simulink model "net"  (R2018a)
settings: Solver=VariableStepAuto  StartTime=0.0  StopTime=10.0  RelTol=1e-3
libraries: neural x115
(part 6 of 6)

== system net/Function Fitting Neural Network/Layer 5/Delays 1 ==
  "p{5}" : Inport  PortDimensions=30
      mask Display: e = 0.06;c1 = [120 230 180]/255;c2 = ([120 230 180]+0)/(256+128);c3 = ([120 230 180]+128)/(256+128);patch([0 1 1 0],[0 0 1 1],c1);patch([0 1 1 1-e 1-e 0+e],[0 0 1 1-e 0+e 0+e],c2);patch([0 0 1 1-e 0+e 0+e],[0 1 1 1-e 1-e 0+e],c3);plot([0 1 1 0 0],[0 0 1 1 0]);
  mux : Mux  Inputs=1
      mask Display: e = 0.06;c1 = [120 150 230]/255;c2 = ([120 150 230]+0)/383;c3 = ([120 150 230]+128)/383;patch([0 1 1 0],[0 0 1 1],c1);patch([0 1 1 1-e 1-e 0+e],[0 0 1 1-e 0+e 0+e],c2);patch([0 0 1 1-e 0+e 0+e],[0 1 1 1-e 1-e 0+e],c3);plot([0 1 1 0 0],[0 0 1 1 0]);disp('Mux')
  "pd{5,4}" : Outport
      mask Display: e = 0.06;c1 = [120 230 180]/255;c2 = ([120 230 180]+0)/(256+128);c3 = ([120 230 180]+128)/(256+128);patch([0 1 1 0],[0 0 1 1],c1);patch([0 1 1 1-e 1-e 0+e],[0 0 1 1-e 0+e 0+e],c2);patch([0 0 1 1-e 0+e 0+e],[0 1 1 1-e 1-e 0+e],c3);plot([0 1 1 0 0],[0 0 1 1 0]);
  wires:
  "p{5}"/1 -> mux/1
  mux/1 -> "pd{5,4}"/1

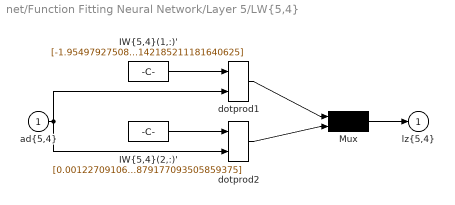
== system net/Function Fitting Neural Network/Layer 5/LW{5,4} ==
  "ad{5,4}" : Inport  PortDimensions=30
      mask Display: e = 0.06;c1 = [120 230 180]/255;c2 = ([120 230 180]+0)/(256+128);c3 = ([120 230 180]+128)/(256+128);patch([0 1 1 0],[0 0 1 1],c1);patch([0 1 1 1-e 1-e 0+e],[0 0 1 1-e 0+e 0+e],c2);patch([0 0 1 1-e 0+e 0+e],[0 1 1 1-e 1-e 0+e],c3);plot([0 1 1 0 0],[0 0 1 1 0]);
  "IW{5,4}(1,:)'" : Constant  Value=[-1.9549792750881287428654786708648316562175750732421875;0.98114975151038585909901712511782534420490264892578125;-0.32675385133424350581066164522781036794185638427734375;-1.93954146076110500729328123270533978939056396484375;0.80033909972648109576454089619801379740238189697265625;-2.975989623557696805988825872191227972507476806640625;-0.2093914166210118221744806987771880812942981719970703125;1.0302617546823376049047737978980876505374908447265625;1.7358886789810872297579180667526088654994964599609375;2.810840906843643072221539114252664148807525634765625;3.216353030282943503692649755976162850856781005859375;1.6089811547340964192898127294029109179973602294921875;-1.1865981966178498208108749167877249419689178466796875;-0.423806008345431306505446400478831492364406585693359375;-1.1447315399113040523815243432181887328624725341796875;0.484091963005052694501983978625503368675708770751953125;4.02934026538351819368699580081738531589508056640625;-1.892775155038552981068278313614428043365478515625;0.0176627926731668417892340272601359174586832523345947265625;-1.93306161386570085625180581700988113880157470703125;2.75222795264777619905771643971092998981475830078125;2.286562436823712740618930183700285851955413818359375;-0.033305608157950757075571601717456360347568988800048828125;2.509966953203996098409334081225097179412841796875;2.29621537725969648846557902288623154163360595703125;1.7190371892103255557771035455516539514064788818359375;-1.5402059024829017896962568556773476302623748779296875;-2.1133202159376711648519631125964224338531494140625;-3.5942783876707107282300057704560458660125732421875;-4.291370172170392294219709583558142185211181640625]
      mask Display: e = 0.06;c1 = [120 150 230]/255;c2 = ([120 150 230]+0)/383;c3 = ([120 150 230]+128)/383;patch([0 1 1 0],[0 0 1 1],c1);patch([0 1 1 1-e 1-e 0+e],[0 0 1 1-e 0+e 0+e],c2);patch([0 0 1 1-e 0+e 0+e],[0 1 1 1-e 1-e 0+e],c3);plot([0 1 1 0 0],[0 0 1 1 0]);disp('weights');
  "IW{5,4}(2,:)'" : Constant  Value=[0.0012270910690294939589251033140726576675660908222198486328125;-0.6810810449990423176558351769926957786083221435546875;-1.3056296010694932174800442226114682853221893310546875;4.19604007762626997021272734489372169264242984354496002197265625e-05;-1.0798036744520616014852976149995811283588409423828125;-0.0003984889985695265024294442479657618605415336787700653076171875;-0.66541233150607104196438967846916057169437408447265625;0.000230191037710248476606811340872127402690239250659942626953125;-0.0002742972495034120780123265692651557401404716074466705322265625;-0.00018045690042486729818931034952100844748201780021190643310546875;-0.0003891359709147802488186929092961463538813404738903045654296875;5.7295766822262235982467226680370231406413950026035308837890625e-05;6.497401433973789826141487235844351744162850081920623779296875e-05;0.0015286228864239315324013990249341077287681400775909423828125;0.000401441358239993544877732833953132285387255251407623291015625;1.3923080293687599695573453573160804808139801025390625;-0.0002824425046101760087245702290914550758316181600093841552734375;2.444007892279712024739823927887982790707610547542572021484375e-05;-0.6811110222253855539520372985862195491790771484375;-0.000382920947363122655439371389007874313392676413059234619140625;-0.000404061427818954246350691139610944446758367121219635009765625;-0.00011397111956974108164242220908590752515010535717010498046875;1.616154737395004037381340822321362793445587158203125;-0.00052263339356889708560427454386854151380248367786407470703125;-0.000254780199442045042663995690901401758310385048389434814453125;-0.0003666521092529675929748422813503339057206176221370697021484375;-4.62947169141729184872226243729897987577714957296848297119140625e-05;7.962574651814685708535457298040682871942408382892608642578125e-05;0.000351625638330074177968775916980348483775742352008819580078125;-0.0002637754488221425385428842158574980203411541879177093505859375]
      mask Display: e = 0.06;c1 = [120 150 230]/255;c2 = ([120 150 230]+0)/383;c3 = ([120 150 230]+128)/383;patch([0 1 1 0],[0 0 1 1],c1);patch([0 1 1 1-e 1-e 0+e],[0 0 1 1-e 0+e 0+e],c2);patch([0 0 1 1-e 0+e 0+e],[0 1 1 1-e 1-e 0+e],c3);plot([0 1 1 0 0],[0 0 1 1 0]);disp('weights');
  Mux : Mux  Inputs=2
      mask Display: e = 0.06;c1 = [120 150 230]/255;c2 = ([120 150 230]+0)/383;c3 = ([120 150 230]+128)/383;patch([0 1 1 0],[0 0 1 1],c1);patch([0 1 1 1-e 1-e 0+e],[0 0 1 1-e 0+e 0+e],c2);patch([0 0 1 1-e 0+e 0+e],[0 1 1 1-e 1-e 0+e],c3);plot([0 1 1 0 0],[0 0 1 1 0]);disp('Mux');
  dotprod1 : neural/Weight Functions/dotprod
  dotprod2 : neural/Weight Functions/dotprod
  "lz{5,4}" : Outport
      mask Display: e = 0.06;c1 = [120 230 180]/255;c2 = ([120 230 180]+0)/(256+128);c3 = ([120 230 180]+128)/(256+128);patch([0 1 1 0],[0 0 1 1],c1);patch([0 1 1 1-e 1-e 0+e],[0 0 1 1-e 0+e 0+e],c2);patch([0 0 1 1-e 0+e 0+e],[0 1 1 1-e 1-e 0+e],c3);plot([0 1 1 0 0],[0 0 1 1 0]);
  wires:
  "IW{5,4}(1,:)'"/1 -> dotprod1/1
  "ad{5,4}"/1 -> dotprod1/2, dotprod2/2
  dotprod1/1 -> Mux/1
  "IW{5,4}(2,:)'"/1 -> dotprod2/1
  dotprod2/1 -> Mux/2
  Mux/1 -> "lz{5,4}"/1
